simulink model "rSOC"  (R2024b)
settings: Solver=FixedStepAuto  StartTime=0.0  StopTime=10.0  RelTol=1e-3  EnableMultiTasking=on
undefined symbols (not defined in the file): EAccumulatorCapacity, QAccumulatorCapacity, tSystemsTask
settings Model: DataDictionary=Master_Dictionary.sldd  EnableAccessToBaseWorkspace=off  Creator=torni  LastModifiedBy=Will
settings OptimizationCC: DefaultParameterBehavior=Inlined  EnhancedBackFolding=on  PassReuseOutputArgsAs=Individual arguments  ZeroExternalMemoryAtStartup=off  ZeroInternalMemoryAtStartup=off  MaxStackSize=8192  OptimizeBlockOrder=speed  DifferentSizesBufferReuse=on  OptimizationCustomize=off  EfficientTunableParamExpr=on
settings DebuggingCC: ParameterTunabilityLossMsg=error
settings HardwareCC: ProdBitPerPointer=32  ProdBitPerSizeT=32  ProdBitPerPtrDiffT=32  ProdLargestAtomicInteger=Long  ProdLargestAtomicFloat=Double  ProdWordSize=32  ProdLongLongMode=on  ProdHWDeviceType=ARM Compatible->ARM Cortex-M
settings SFSimCC: MATLABDynamicMemAlloc=off
settings RTWCC: Description=Embedded Coder  SystemTargetFile=ert.tlc  HardwareBoard=STM32H7xx Based (Single-core)  TemplateMakefile=ert_default_tmf  Toolchain=GNU Tools for ARM Embedded Processors
settings CodeAppCC: ForceParamTrailComments=on  IgnoreCustomStorageClasses=off  OperatorAnnotations=on  SimulinkDataObjDesc=on  SFDataObjDesc=on  InsertBlockDesc=on
settings ERTTargetCC: TargetLangStandard=C99 (ISO)  CodeReplacementLibrary=ARM Cortex-M  ExtModeTransport=3  ExtModeStaticAlloc=on  ExtModeStaticAllocSize=2048  ExtModeMexFile=ext_xcp  ExtModeIntrfLevel=Level2 - Open

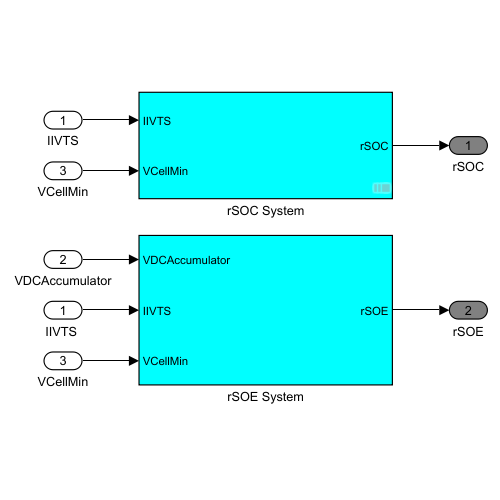
[thumbnail: Simulink's stored preview of the top-level diagram]
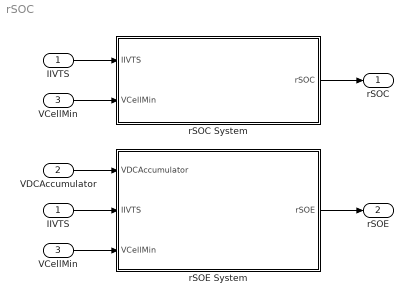
== system rSOC ==
  IIVTS : Inport  OutDataTypeStr=double
  VDCAccumulator : Inport  Port=2  OutDataTypeStr=double
  VCellMin : Inport  Port=3  OutDataTypeStr=double
  "IIVTS " : InportShadow  OutDataTypeStr=double
  "VCellMin " : InportShadow  Port=3  OutDataTypeStr=double
  rSOC System : Subsystem
  rSOE System : Subsystem
  rSOC : Outport  OutDataTypeStr=double  VectorParamsAs1DForOutWhenUnconnected=off
  rSOE : Outport  Port=2  OutDataTypeStr=double  VectorParamsAs1DForOutWhenUnconnected=off
  wires:
  "VCellMin "/1 -> rSOE System/3(VCellMin)
  VCellMin/1 -> rSOC System/2(VCellMin)
  rSOC System/1(rSOC) -> rSOC/1
  IIVTS/1 -> rSOC System/1(IIVTS)
  rSOE System/1(rSOE) -> rSOE/1
  VDCAccumulator/1 -> rSOE System/1(VDCAccumulator)
  "IIVTS "/1 -> rSOE System/2(IIVTS)

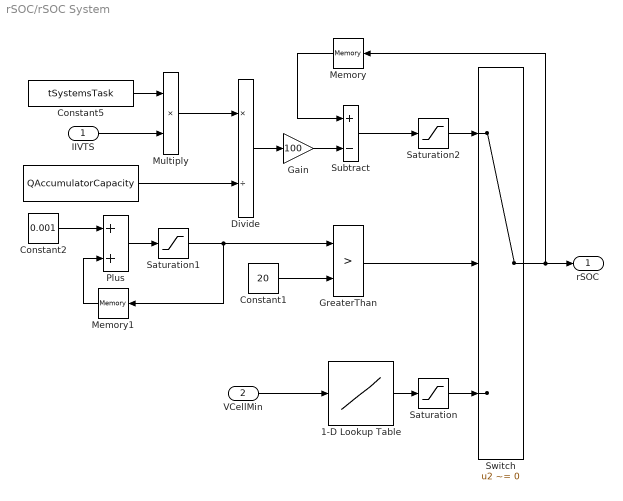
== system rSOC/rSOC System ==
  IIVTS : Inport  OutDataTypeStr=double
  VCellMin : Inport  Port=2  OutDataTypeStr=double
  " " : Constant  Value=QAccumulatorCapacity  SampleTime=-1
  1-D Lookup Table : Lookup_n-D  NumberOfTableDimensions=1  BreakpointsForDimension1=[2.748915,2.809015,2.871858,2.926176,2.975664,3.020264,3.060799,3.096421,3.129003,3.15873,3.184746,3.209297,3.228753,3.248677,3.266712,3.282122,3.298795,3.313867,3.327881,3.340033,3.353216,3.365912,3.377531,3.388307,3.397827,3.409236,3.41903,3.428383,3.437904,3.446442,3.455239,3.463243,3.471737,3.478276,3.487228,3.493993,3.500748,3.507915,3.51485,3.521746,3.527677,3.534373,3.540189,3.545965,3.552474,3.557842,3.563178,3.569147,3.574396,3.579599,3.585067,3.58998,3.594202,3.600052,3.603192,3.608541,3.61328,3.61768,3.620936,3.626256,3.630339,3.634081,3.638963,3.641832,3.64574,3.649164,3.652797,3.656277,3.658721,3.662538,3.6644,3.667905,3.669343,3.671838,3.673092,3.674846,3.67656,3.676797,3.677382,3.678427,3.678977,3.68049,3.680723,3.680768,3.681006,3.68259,3.682729,3.683128,3.683577,3.683754,3.683877,3.684147,3.684647,3.684693,3.684885,3.685473,3.685729,3.68575,3.685814,3.685833,3.686373,3.68659,3.686594,3.687267,3.687637,3.687693,3.68776,3.68794,3.688069,3.688098,3.68827,3.688355,3.688605,3.68886,3.689126,3.689227,3.689307,3.689353,3.689826,3.690051,3.690098,3.690209,3.690429,3.690553,3.690744,3.690913,3.69101,3.691391,3.691544,3.691776,3.691864,3.692156,3.692534,3.692807,3.693429,3.693614,3.693921,3.695275,3.696163,3.696393,3.697229,3.697912,3.699352,3.700633,3.701149,3.702371,3.703016,3.703865,3.704813,3.705691,3.706607,3.707544,3.707747,3.707797,3.709272,3.709388,3.710816,3.71096,3.711942,3.712774,3.712801,3.713666,3.714181,3.714663,3.715938,3.716274,3.716611,3.718012,3.718626,3.718696,3.719342,3.720962,3.721146,3.722235,3.722854,3.72288,3.723581,3.724416,3.725047,3.726079,3.726948,3.727513,3.728574,3.728695,3.729848,3.730034,3.731323,3.7325,3.732953,3.733126,3.733288,3.734068,3.734226,3.736014,3.736465,3.737267,3.73808,3.738637,3.738805,3.739934,3.740268,3.74099,3.741444,3.741951,3.742475,3.743142,3.744253,3.744821,3.745328,3.746031,3.746108,3.746411,3.746735,3.747394,3.747694,3.747987,3.74917,3.749943,3.750428,3.750979,3.751274,3.751692,3.751729,3.753137,3.753762,3.754916,3.755108,3.755369,3.75605,3.756547,3.757696,3.757798,3.758395,3.758849,3.759869,3.760056,3.760583,3.760602,3.761209,3.762449,3.763372,3.763899,3.764629,3.764888,3.764908,3.766136,3.766225,3.767197,3.767809,3.768881,3.769684,3.770029,3.770277,3.771483,3.771535,3.771977,3.773375,3.773672,3.774066,3.775319,3.776238,3.776252,3.776357,3.776759,3.777201,3.778331,3.778653,3.778826,3.779734,3.780663,3.780888,3.782299,3.782827,3.783843,3.783858,3.784073,3.785269,3.785463,3.786895,3.787937,3.7883,3.788515,3.788785,3.789686,3.789772,3.791175,3.791728,3.792205,3.792721,3.793107,3.794563,3.794655,3.795103,3.795634,3.795679,3.796772,3.79774,3.79787,3.798018,3.799034,3.799197,3.800229,3.800703,3.801729,3.801952,3.802736,3.803337,3.803792,3.804584,3.804868,3.805291,3.805557,3.805716,3.807394,3.807866,3.808174,3.808544,3.808641,3.810184,3.810437,3.810741,3.810916,3.811353,3.811592,3.812781,3.812937,3.813645,3.814436,3.814518,3.814871,3.815779,3.816737,3.817061,3.81798,3.817991,3.818514,3.81956,3.819601,3.820385,3.820473,3.820727,3.821853,3.822421,3.823027,3.823103,3.823858,3.823914,3.824189,3.824797,3.826264,3.826363,3.82722,3.827358,3.8279,3.828673,3.829267,3.830035,3.830086,3.830693,3.831,3.831393,3.83181,3.832862,3.833375,3.833491,3.834954,3.835561,3.836034,3.836307,3.836421,3.83748,3.838628,3.838905,3.839045,3.839335,3.839621,3.840702,3.841288,3.841565,3.842478,3.842707,3.843615,3.844414,3.8451,3.845431,3.845546,3.846635,3.847116,3.8476,3.848104,3.849007,3.849122,3.850736,3.850973,3.851686,3.852313,3.85252,3.853628,3.853738,3.85419,3.854674,3.856088,3.856272,3.857083,3.857089,3.857699,3.858152,3.859015,3.860705,3.86082,3.860984,3.861649,3.86242,3.862958,3.863578,3.863696,3.864094,3.865429,3.86582,3.867116,3.86728,3.867942,3.868924,3.869488,3.869759,3.870872,3.870923,3.87186,3.87269,3.873231,3.874437,3.874703,3.875682,3.876338,3.876782,3.877167,3.878466,3.878653,3.878835,3.880832,3.88088,3.881641,3.881976,3.883348,3.883358,3.884452,3.884504,3.886708,3.886981,3.887415 ...(+4304 chars)]  Table=[0,0.082641158,0.189757207,0.296975661,0.40409171,0.511207759,0.618323808,0.725337451,0.8324535,0.939569549,1.046583193,1.153699241,1.26081529,1.367828934,1.474944983,1.582061032,1.689074675,1.796190724,1.903306773,2.010422822,2.117538871,2.224552514,2.331668563,2.438682206,2.545798255,2.653016709,2.760132758,2.867146402,2.974160045,3.081173689,3.188392143,3.295405787,3.40241943,3.509433073,3.616446717,3.72346036,3.830474004,3.937487647,4.044501291,4.151412529,4.258426172,4.365542221,4.472555865,4.579569508,4.686583152,4.793596795,4.900610439,5.007931298,5.114944942,5.221958585,5.328972229,5.436088278,5.543101921,5.65021797,5.75753883,5.864552473,5.971668522,6.078682165,6.185695809,6.292811858,6.399927907,6.507043955,6.614057599,6.721173648,6.828187291,6.935200935,7.042214578,7.149228222,7.256241865,7.363357914,7.470473963,7.577487606,7.68450125,7.791514893,7.898528537,8.00554218,8.112658229,8.219671873,8.326787921,8.540917614,8.433801565,8.647931257,8.862163355,8.755047306,8.969279404,9.076497858,9.183511502,9.397641194,9.290627551,9.825798173,9.504654837,9.611668481,10.03992787,9.71878453,9.932914222,10.3609688,10.57499608,10.25395515,10.46798244,10.14694151,11.00335787,10.78933059,10.68221454,10.89634423,11.11047392,11.752863,11.21748757,11.9670951,11.3243988,11.43161726,11.64554214,11.5386309,11.86008145,12.07410874,12.28803362,12.18112238,12.93032029,12.50216331,12.60917696,12.7161906,12.39504727,12.82330665,13.03733394,13.25136122,13.14434758,13.35847727,13.6795182,13.46549092,13.57250456,14.00066154,13.89354549,13.78653185,14.10767518,14.21468883,14.42892092,14.32180487,14.53593457,14.64294821,14.75006426,14.96409155,14.8570779,15.07110519,15.17852845,15.2855421,15.39265815,15.49967179,15.60668543,15.71369908,15.82081513,15.92782877,16.03494482,16.14185606,16.2488697,16.35588334,16.46299939,16.57001304,16.67712909,16.78424513,16.89125878,17.21240211,16.99837483,17.10538847,17.42673662,17.31972297,17.53375026,17.74787995,17.64086631,17.854996,18.17603693,17.96200964,18.06912569,18.28305057,18.39006422,18.49707786,18.60409151,18.71110515,18.81811879,18.92513244,19.03214608,19.13915972,19.24617337,19.35318701,19.46030306,19.5673167,19.67422794,19.78124158,19.88825523,20.10248732,19.99537128,20.20950097,20.5305419,20.42352826,20.31661702,20.63755554,20.74456919,20.85178764,20.95900609,21.06612214,21.17313579,21.28014943,21.38726548,21.49438153,21.60139517,21.70851122,21.92253851,21.81552486,22.02955215,22.13687301,22.24388665,22.45791394,22.3509003,22.56492758,22.99298216,22.67194123,22.88596851,22.77895487,23.0999958,23.20711185,23.31412549,23.42124154,23.63526883,23.52825519,23.74228247,23.84929612,24.17054186,24.06342581,23.95620735,24.2775555,24.38477396,24.59890365,24.81323815,24.7061221,24.4917876,24.92025179,25.02716303,25.13417668,25.45542242,25.24108791,25.34851118,25.56243606,25.6694497,25.77646335,25.88378421,26.09781149,25.99079785,26.20482514,26.31183878,26.41895483,26.52617328,26.63339174,26.74030298,26.84731662,26.95422786,27.06134391,27.27567841,27.16835755,27.38269205,27.59671934,27.4897057,27.70363058,28.02528594,27.81064422,27.9182723,28.13219718,28.23921082,28.45323811,28.34612206,28.56025175,28.6672654,28.77427904,28.88129268,28.98830633,29.09531997,29.20243602,29.41666812,29.30944966,29.630593,29.52357936,29.73770905,29.84472269,30.05874998,29.95173633,30.16576362,30.27277727,30.3796885,30.48680455,30.5938182,30.80774308,30.70072943,30.91465432,31.02166796,31.23569525,31.1285792,31.34260648,31.44962013,31.55653137,31.87746989,31.66354501,31.77045625,31.98489316,32.0919068,32.30593409,32.19892044,32.41294773,32.51985897,32.62687261,32.73388625,32.8408999,32.94781114,33.05482478,33.16183842,33.37596812,33.26885207,33.5899954,33.48298176,33.69772588,33.80463712,34.01886922,33.91175317,34.44682139,34.12588286,34.2327941,34.33980774,34.55403984,34.76816953,34.66105349,34.87508077,34.98219682,35.19694095,35.08941528,35.30405699,35.41096823,35.51787947,35.62499552,35.73200916,35.83922762,35.94624126 ...(+7104 chars)]  InternalRulePriority=Speed  RndMeth=Simplest
  Constant1 : Constant  Value=20  SampleTime=-1
  Constant2 : Constant  Value=0.001  SampleTime=-1
  Constant5 : Constant  Value=tSystemsTask  SampleTime=-1
  Divide : Product  Inputs=*/
  Gain : Gain  Gain=100
  GreaterThan : RelationalOperator  Operator=>  OutDataTypeStr=boolean  RndMeth=Simplest  InputSameDT=off
  Memory : Memory  InitialCondition=100  InheritSampleTime=on
  Memory1 : Memory  InheritSampleTime=on
  Multiply : Product
  Plus : Sum
  Saturation : Saturate  UpperLimit=100  LowerLimit=0
  Saturation1 : Saturate  UpperLimit=25  LowerLimit=0
  Saturation2 : Saturate  UpperLimit=100  LowerLimit=0
  Subtract : Sum  Inputs=+-
  Switch : Switch  Criteria=u2 ~= 0  Threshold=20  SaturateOnIntegerOverflow=off  InputSameDT=off
  rSOC : Outport  OutDataTypeStr=double  VectorParamsAs1DForOutWhenUnconnected=off
  wires:
  Memory/1 -> Subtract/1
  Constant5/1 -> Multiply/1
  IIVTS/1 -> Multiply/2
  Multiply/1 -> Divide/1
  Divide/1 -> Gain/1
  " "/1 -> Divide/2
  Gain/1 -> Subtract/2
  VCellMin/1 -> 1-D Lookup Table/1
  Subtract/1 -> Saturation2/1
  Switch/1 -> Memory/1, rSOC/1
  1-D Lookup Table/1 -> Saturation/1
  Constant2/1 -> Plus/1
  Memory1/1 -> Plus/2
  GreaterThan/1 -> Switch/2
  Plus/1 -> Saturation1/1
  Saturation1/1 -> Memory1/1, GreaterThan/1
  Constant1/1 -> GreaterThan/2
  Saturation/1 -> Switch/3
  Saturation2/1 -> Switch/1

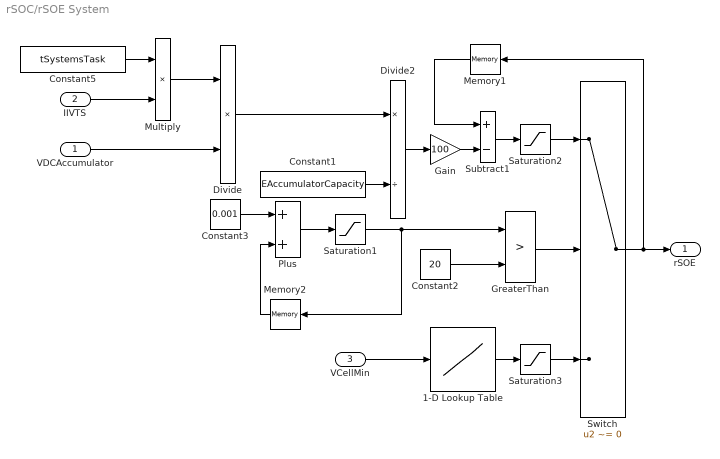
== system rSOC/rSOE System ==
  VDCAccumulator : Inport  OutDataTypeStr=double
  IIVTS : Inport  Port=2  OutDataTypeStr=double
  VCellMin : Inport  Port=3  OutDataTypeStr=double
  1-D Lookup Table : Lookup_n-D  NumberOfTableDimensions=1  BreakpointsForDimension1=[2.748915,2.809015,2.871858,2.926176,2.975664,3.020264,3.060799,3.096421,3.129003,3.15873,3.184746,3.209297,3.228753,3.248677,3.266712,3.282122,3.298795,3.313867,3.327881,3.340033,3.353216,3.365912,3.377531,3.388307,3.397827,3.409236,3.41903,3.428383,3.437904,3.446442,3.455239,3.463243,3.471737,3.478276,3.487228,3.493993,3.500748,3.507915,3.51485,3.521746,3.527677,3.534373,3.540189,3.545965,3.552474,3.557842,3.563178,3.569147,3.574396,3.579599,3.585067,3.58998,3.594202,3.600052,3.603192,3.608541,3.61328,3.61768,3.620936,3.626256,3.630339,3.634081,3.638963,3.641832,3.64574,3.649164,3.652797,3.656277,3.658721,3.662538,3.6644,3.667905,3.669343,3.671838,3.673092,3.674846,3.67656,3.676797,3.677382,3.678427,3.678977,3.68049,3.680723,3.680768,3.681006,3.68259,3.682729,3.683128,3.683577,3.683754,3.683877,3.684147,3.684647,3.684693,3.684885,3.685473,3.685729,3.68575,3.685814,3.685833,3.686373,3.68659,3.686594,3.687267,3.687637,3.687693,3.68776,3.68794,3.688069,3.688098,3.68827,3.688355,3.688605,3.68886,3.689126,3.689227,3.689307,3.689353,3.689826,3.690051,3.690098,3.690209,3.690429,3.690553,3.690744,3.690913,3.69101,3.691391,3.691544,3.691776,3.691864,3.692156,3.692534,3.692807,3.693429,3.693614,3.693921,3.695275,3.696163,3.696393,3.697229,3.697912,3.699352,3.700633,3.701149,3.702371,3.703016,3.703865,3.704813,3.705691,3.706607,3.707544,3.707747,3.707797,3.709272,3.709388,3.710816,3.71096,3.711942,3.712774,3.712801,3.713666,3.714181,3.714663,3.715938,3.716274,3.716611,3.718012,3.718626,3.718696,3.719342,3.720962,3.721146,3.722235,3.722854,3.72288,3.723581,3.724416,3.725047,3.726079,3.726948,3.727513,3.728574,3.728695,3.729848,3.730034,3.731323,3.7325,3.732953,3.733126,3.733288,3.734068,3.734226,3.736014,3.736465,3.737267,3.73808,3.738637,3.738805,3.739934,3.740268,3.74099,3.741444,3.741951,3.742475,3.743142,3.744253,3.744821,3.745328,3.746031,3.746108,3.746411,3.746735,3.747394,3.747694,3.747987,3.74917,3.749943,3.750428,3.750979,3.751274,3.751692,3.751729,3.753137,3.753762,3.754916,3.755108,3.755369,3.75605,3.756547,3.757696,3.757798,3.758395,3.758849,3.759869,3.760056,3.760583,3.760602,3.761209,3.762449,3.763372,3.763899,3.764629,3.764888,3.764908,3.766136,3.766225,3.767197,3.767809,3.768881,3.769684,3.770029,3.770277,3.771483,3.771535,3.771977,3.773375,3.773672,3.774066,3.775319,3.776238,3.776252,3.776357,3.776759,3.777201,3.778331,3.778653,3.778826,3.779734,3.780663,3.780888,3.782299,3.782827,3.783843,3.783858,3.784073,3.785269,3.785463,3.786895,3.787937,3.7883,3.788515,3.788785,3.789686,3.789772,3.791175,3.791728,3.792205,3.792721,3.793107,3.794563,3.794655,3.795103,3.795634,3.795679,3.796772,3.79774,3.79787,3.798018,3.799034,3.799197,3.800229,3.800703,3.801729,3.801952,3.802736,3.803337,3.803792,3.804584,3.804868,3.805291,3.805557,3.805716,3.807394,3.807866,3.808174,3.808544,3.808641,3.810184,3.810437,3.810741,3.810916,3.811353,3.811592,3.812781,3.812937,3.813645,3.814436,3.814518,3.814871,3.815779,3.816737,3.817061,3.81798,3.817991,3.818514,3.81956,3.819601,3.820385,3.820473,3.820727,3.821853,3.822421,3.823027,3.823103,3.823858,3.823914,3.824189,3.824797,3.826264,3.826363,3.82722,3.827358,3.8279,3.828673,3.829267,3.830035,3.830086,3.830693,3.831,3.831393,3.83181,3.832862,3.833375,3.833491,3.834954,3.835561,3.836034,3.836307,3.836421,3.83748,3.838628,3.838905,3.839045,3.839335,3.839621,3.840702,3.841288,3.841565,3.842478,3.842707,3.843615,3.844414,3.8451,3.845431,3.845546,3.846635,3.847116,3.8476,3.848104,3.849007,3.849122,3.850736,3.850973,3.851686,3.852313,3.85252,3.853628,3.853738,3.85419,3.854674,3.856088,3.856272,3.857083,3.857089,3.857699,3.858152,3.859015,3.860705,3.86082,3.860984,3.861649,3.86242,3.862958,3.863578,3.863696,3.864094,3.865429,3.86582,3.867116,3.86728,3.867942,3.868924,3.869488,3.869759,3.870872,3.870923,3.87186,3.87269,3.873231,3.874437,3.874703,3.875682,3.876338,3.876782,3.877167,3.878466,3.878653,3.878835,3.880832,3.88088,3.881641,3.881976,3.883348,3.883358,3.884452,3.884504,3.886708,3.886981,3.887415 ...(+4304 chars)]  Table=[0,0.082641158,0.189757207,0.296975661,0.40409171,0.511207759,0.618323808,0.725337451,0.8324535,0.939569549,1.046583193,1.153699241,1.26081529,1.367828934,1.474944983,1.582061032,1.689074675,1.796190724,1.903306773,2.010422822,2.117538871,2.224552514,2.331668563,2.438682206,2.545798255,2.653016709,2.760132758,2.867146402,2.974160045,3.081173689,3.188392143,3.295405787,3.40241943,3.509433073,3.616446717,3.72346036,3.830474004,3.937487647,4.044501291,4.151412529,4.258426172,4.365542221,4.472555865,4.579569508,4.686583152,4.793596795,4.900610439,5.007931298,5.114944942,5.221958585,5.328972229,5.436088278,5.543101921,5.65021797,5.75753883,5.864552473,5.971668522,6.078682165,6.185695809,6.292811858,6.399927907,6.507043955,6.614057599,6.721173648,6.828187291,6.935200935,7.042214578,7.149228222,7.256241865,7.363357914,7.470473963,7.577487606,7.68450125,7.791514893,7.898528537,8.00554218,8.112658229,8.219671873,8.326787921,8.540917614,8.433801565,8.647931257,8.862163355,8.755047306,8.969279404,9.076497858,9.183511502,9.397641194,9.290627551,9.825798173,9.504654837,9.611668481,10.03992787,9.71878453,9.932914222,10.3609688,10.57499608,10.25395515,10.46798244,10.14694151,11.00335787,10.78933059,10.68221454,10.89634423,11.11047392,11.752863,11.21748757,11.9670951,11.3243988,11.43161726,11.64554214,11.5386309,11.86008145,12.07410874,12.28803362,12.18112238,12.93032029,12.50216331,12.60917696,12.7161906,12.39504727,12.82330665,13.03733394,13.25136122,13.14434758,13.35847727,13.6795182,13.46549092,13.57250456,14.00066154,13.89354549,13.78653185,14.10767518,14.21468883,14.42892092,14.32180487,14.53593457,14.64294821,14.75006426,14.96409155,14.8570779,15.07110519,15.17852845,15.2855421,15.39265815,15.49967179,15.60668543,15.71369908,15.82081513,15.92782877,16.03494482,16.14185606,16.2488697,16.35588334,16.46299939,16.57001304,16.67712909,16.78424513,16.89125878,17.21240211,16.99837483,17.10538847,17.42673662,17.31972297,17.53375026,17.74787995,17.64086631,17.854996,18.17603693,17.96200964,18.06912569,18.28305057,18.39006422,18.49707786,18.60409151,18.71110515,18.81811879,18.92513244,19.03214608,19.13915972,19.24617337,19.35318701,19.46030306,19.5673167,19.67422794,19.78124158,19.88825523,20.10248732,19.99537128,20.20950097,20.5305419,20.42352826,20.31661702,20.63755554,20.74456919,20.85178764,20.95900609,21.06612214,21.17313579,21.28014943,21.38726548,21.49438153,21.60139517,21.70851122,21.92253851,21.81552486,22.02955215,22.13687301,22.24388665,22.45791394,22.3509003,22.56492758,22.99298216,22.67194123,22.88596851,22.77895487,23.0999958,23.20711185,23.31412549,23.42124154,23.63526883,23.52825519,23.74228247,23.84929612,24.17054186,24.06342581,23.95620735,24.2775555,24.38477396,24.59890365,24.81323815,24.7061221,24.4917876,24.92025179,25.02716303,25.13417668,25.45542242,25.24108791,25.34851118,25.56243606,25.6694497,25.77646335,25.88378421,26.09781149,25.99079785,26.20482514,26.31183878,26.41895483,26.52617328,26.63339174,26.74030298,26.84731662,26.95422786,27.06134391,27.27567841,27.16835755,27.38269205,27.59671934,27.4897057,27.70363058,28.02528594,27.81064422,27.9182723,28.13219718,28.23921082,28.45323811,28.34612206,28.56025175,28.6672654,28.77427904,28.88129268,28.98830633,29.09531997,29.20243602,29.41666812,29.30944966,29.630593,29.52357936,29.73770905,29.84472269,30.05874998,29.95173633,30.16576362,30.27277727,30.3796885,30.48680455,30.5938182,30.80774308,30.70072943,30.91465432,31.02166796,31.23569525,31.1285792,31.34260648,31.44962013,31.55653137,31.87746989,31.66354501,31.77045625,31.98489316,32.0919068,32.30593409,32.19892044,32.41294773,32.51985897,32.62687261,32.73388625,32.8408999,32.94781114,33.05482478,33.16183842,33.37596812,33.26885207,33.5899954,33.48298176,33.69772588,33.80463712,34.01886922,33.91175317,34.44682139,34.12588286,34.2327941,34.33980774,34.55403984,34.76816953,34.66105349,34.87508077,34.98219682,35.19694095,35.08941528,35.30405699,35.41096823,35.51787947,35.62499552,35.73200916,35.83922762,35.94624126 ...(+7104 chars)]  InternalRulePriority=Speed  RndMeth=Simplest
  Constant1 : Constant  Value=EAccumulatorCapacity  SampleTime=-1
  Constant2 : Constant  Value=20  SampleTime=-1
  Constant3 : Constant  Value=0.001  SampleTime=-1
  Constant5 : Constant  Value=tSystemsTask  SampleTime=-1
  Divide : Product  Inputs=**
  Divide2 : Product  Inputs=*/
  Gain : Gain  Gain=100
  GreaterThan : RelationalOperator  Operator=>  OutDataTypeStr=boolean  RndMeth=Simplest  InputSameDT=off
  Memory1 : Memory  InitialCondition=100  InheritSampleTime=on
  Memory2 : Memory  InheritSampleTime=on
  Multiply : Product
  Plus : Sum
  Saturation1 : Saturate  UpperLimit=25  LowerLimit=0
  Saturation2 : Saturate  UpperLimit=100  LowerLimit=0
  Saturation3 : Saturate  UpperLimit=100  LowerLimit=0
  Subtract1 : Sum  Inputs=+-
  Switch : Switch  Criteria=u2 ~= 0  SaturateOnIntegerOverflow=off  InputSameDT=off
  rSOE : Outport  OutDataTypeStr=double  VectorParamsAs1DForOutWhenUnconnected=off
  wires:
  VDCAccumulator/1 -> Divide/2
  Divide/1 -> Divide2/1
  Divide2/1 -> Gain/1
  Memory1/1 -> Subtract1/1
  Subtract1/1 -> Saturation2/1
  Constant5/1 -> Multiply/1
  Multiply/1 -> Divide/1
  IIVTS/1 -> Multiply/2
  Constant1/1 -> Divide2/2
  Gain/1 -> Subtract1/2
  1-D Lookup Table/1 -> Saturation3/1
  VCellMin/1 -> 1-D Lookup Table/1
  Switch/1 -> Memory1/1, rSOE/1
  Constant3/1 -> Plus/1
  Memory2/1 -> Plus/2
  GreaterThan/1 -> Switch/2
  Saturation1/1 -> Memory2/1, GreaterThan/1
  Plus/1 -> Saturation1/1
  Constant2/1 -> GreaterThan/2
  Saturation2/1 -> Switch/1
  Saturation3/1 -> Switch/3
